simulink library "tqd"  (R2021b)
settings: Solver=VariableStepAuto  StartTime=0.0  StopTime=10.0  RelTol=1e-3
undefined symbols (not defined in the file): ATQD_AfterTqMinGain_X_Deg, ATQD_APSCreepBaseTqD_X_kph, ATQD_APSCreepBaseTqD_Y_Deg, ATQD_APSCreepBaseTqR_X_kph, ATQD_APSCreepBaseTqR_Y_Deg, ATQD_APSCreepIterm_X_kph, ATQD_APSCreepIterm_Y_kph, ATQD_APSCreepPterm_X_kph, ATQD_APSCreepPterm_Y_kph, ATQD_APSDecReq_X_kph, ATQD_APSDecReq_Y_mps2, ATQD_APSDecReqCMD_X_kph, ATQD_APSDecReqTs_X_pct, ATQD_APSDecTimeGain_X_Deg, ATQD_APSDecTimeGain_Y_s, ATQD_APSReqLowSpd_X_Deg, ATQD_AutoHoldReleaseBPS_X_Deg, ATQD_AWDLoadTrqnsGain_X_kg, ATQD_AWDLoadTrqnsGain_Y_pct, ATQD_BOSEnBPSPosn_X_kph, ATQD_BOSMap_X_rpm, ATQD_BOSMap_Y_pct, ATQD_CreepBaseTqD_X_kph, ATQD_CreepBaseTqD_Y_Deg, ATQD_CreepBaseTqR_X_kph, ATQD_CreepBaseTqR_Y_Deg, ATQD_CreepBPSDisPosn_X_Deg, ATQD_CreepBPSDisPosnR_X_Deg, ATQD_CreepBPSEnPosn_X_Deg, ATQD_CreepBPSEnPosnR_X_Deg, ATQD_CreepDeltaTq_X_kph, ATQD_CreepIterm_X_kph, ATQD_CreepIterm_Y_kph, ATQD_CreepItermMaxLimit_X_pct, ATQD_CreepPreloadTime_X_kph, ATQD_CreepPreloadTq_X_kph, ATQD_CreepPreloadTq_Y_s, ATQD_CreepProtTq_X_Deg, ATQD_CreepPterm_X_kph, ATQD_CreepPterm_Y_kph, ATQD_CreepRrTqSpRat_X_rpm, ATQD_CreepRrTqSpRat_Y_Nm, ATQD_CreepTargetSpdD_X_pct, ATQD_CreepTargetSpdR_X_pct, ATQD_ECOTqMapD_X_rpm, ATQD_ECOTqMapD_Y_pct, ATQD_EMTqMapD_X_rpm, ATQD_EMTqMapD_Y_pct, ATQD_EOPDTqMapDCon_X_rpm, ATQD_EOPDTqMapDCon_Y_Deg, ATQD_EscapeModePedTq_X_pct, ATQD_EscapeModePedTq_Y_rpm, ATQD_EscapeModePedTqFr_X_pct, ATQD_EscapeModePedTqFr_Y_rpm, ATQD_EstInitVehWeight_X_c, ATQD_FAfterTqCMDGain_X_rpm, ATQD_FAfterTqCMDGain_Y_pct, ATQD_FrLossMAPLowV_X_rpm, ATQD_FrLossMAPLowV_Y_Nm, ATQD_FrMotActReduce_X_rpm ... (+772)
libraries: simulink x211, hcu_lib x179, tqr x3
(part 2 of 28)

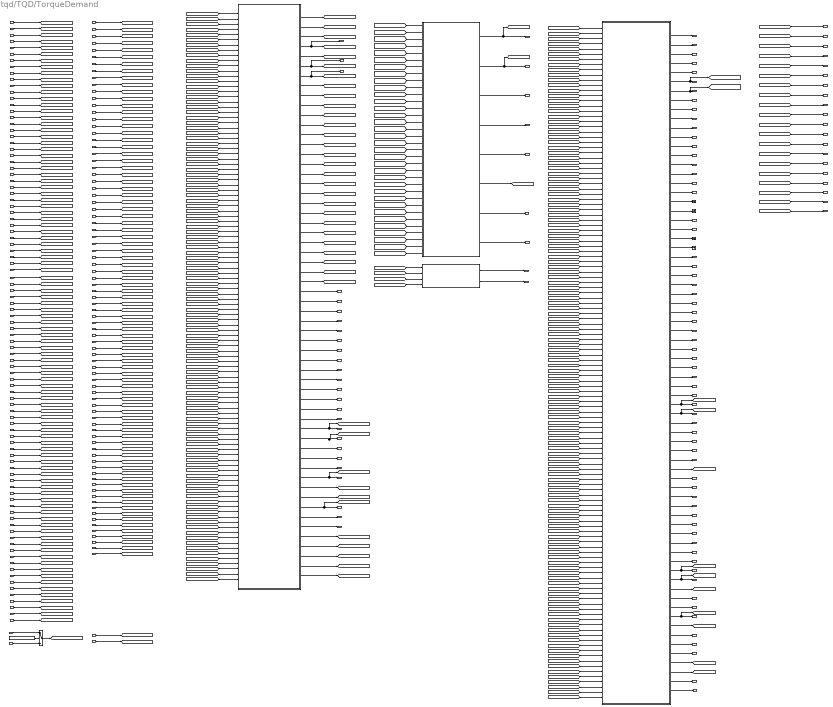
== system tqd/TQD/TorqueDemand ==
  note: Input Signals
  task_time_s : Inport
  VDHP_ActAPSPosn_pct : Inport  Port=2
  VDHP_LowIdleAccPedal_flg : Inport  Port=3
  VPMM_PowerSta_enum : Inport  Port=4
  VPMM_DrivetrainSelect_enum : Inport  Port=5
  VPMM_SysPowerMode_enum : Inport  Port=6
  VINP_VehSpeed_kph : Inport  Port=7
  VINP_BrkSwSta_flg : Inport  Port=8
  VINP_BrkSwV_flg : Inport  Port=9
  VINP_BrkPedalPos_pct : Inport  Port=10
  VINP_BrkPedalPosSta_flg : Inport  Port=11
  VINP_FrPTCSActive_flg : Inport  Port=12
  VINP_RrPTCSActive_flg : Inport  Port=13
  VINP_FrntAxlTrqReqDrv_Nm : Inport  Port=14
  VINP_RearAxlTrqReqDrv_Nm : Inport  Port=15
  VINP_FrRBCActive_flg : Inport  Port=16
  VINP_RrRBCActive_flg : Inport  Port=17
  VINP_FrntAxlTrqReqBrk_Nm : Inport  Port=18
  VINP_RearAxlTrqReqBrk_Nm : Inport  Port=19
  VINP_CrashOutputSts_enum : Inport  Port=20
  VINP_LongAccel_Gps : Inport  Port=21
  VINP_EPBCarWashMode_flg : Inport  Port=22
  VINP_EPBErrSta_enum : Inport  Port=23
  VINP_EPBSta_enum : Inport  Port=24
  VINP_DOASta_flg : Inport  Port=25
  VINP_GRADE_Deg : Inport  Port=26
  VINP_HSAActive_flg : Inport  Port=27
  VINP_DriverSeatBeltCmd_flg : Inport  Port=28
  VINP_AVHActive_flg : Inport  Port=29
  VINP_PsngrSeatBeltCmd_flg : Inport  Port=30
  VINP_RDriverSeatBeltCmd_flg : Inport  Port=31
  VINP_RCenterSeatBeltCmd_flg : Inport  Port=32
  VINP_RPsngrSeatBeltCmd_flg : Inport  Port=33
  VINP_YawRate_degps : Inport  Port=34
  VINP_SASAngle_Deg : Inport  Port=35
  VINP_ESCActive_flg : Inport  Port=36
  VINP_ABSActive_flg : Inport  Port=37
  VINP_LFRawWhlSpeed_kph : Inport  Port=38
  VINP_LRRawWhlSpeed_kph : Inport  Port=39
  VINP_RFRawWhlSpeed_kph : Inport  Port=40
  VINP_RRRawWhlSpeed_kph : Inport  Port=41
  VINP_ESCOFFStatus_enum : Inport  Port=42
  VINP_IVIPWModeReq_enum : Inport  Port=43
  VINP_IVICreepSWReq_flg : Inport  Port=44
  VINP_RollModeSWCmd_enum : Inport  Port=45
  VINP_IVIPwrLockSW_enum : Inport  Port=46
  VINP_IVIISAOffsetSpd_enum : Inport  Port=47
  VINP_Distanceunit_flg : Inport  Port=48
  VINP_SmartEcoModeSW_flg : Inport  Port=49
  VINP_IVISnowModeCmd_flg : Inport  Port=50
  VINP_IVIACCAdaptiveSta_flg : Inport  Port=51
  VINP_IVITrailerModeSWSta_flg : Inport  Port=52
  VINP_ShifterHandleCmd_enum : Inport  Port=53
  VINP_HVBPwrAvailDchrg_kw : Inport  Port=54
  VINP_HVBPwrAvailChrg_kw : Inport  Port=55
  VINP_HVBattErr_flg : Inport  Port=56
  VINP_DCDCFaultSta_enum : Inport  Port=57
  VINP_ChrgPlugSta_enum : Inport  Port=58
  VINP_HVBattSOC_pct : Inport  Port=59
  VINP_HVBattSOCDis_pct : Inport  Port=60
  VINP_HVBMTempMax_C : Inport  Port=61
  VINP_HVBMTempMin_C : Inport  Port=62
  VINP_ShifterFailsta_enum : Inport  Port=63
  VINP_FrEDURotateDirction_enum : Inport  Port=64
  VINP_RrEDURotateDirction_enum : Inport  Port=65
  VINP_FrTMSpd_RPM : Inport  Port=66
  VINP_RrTMSpd_RPM : Inport  Port=67
  VINP_FrRegenAvailTq_Nm : Inport  Port=68
  VINP_RrRegenAvailTq_Nm : Inport  Port=69
  VINP_FrEDURealTMTq_Nm : Inport  Port=70
  VINP_RrEDURealTMTq_Nm : Inport  Port=71
  VINP_FrMotorAvailTq_Nm : Inport  Port=72
  VINP_RrMotorAvailTq_Nm : Inport  Port=73
  VINP_MCUWarnF_enum : Inport  Port=74
  VINP_MCUWarnR_enum : Inport  Port=75
  VINP_FrMCUDCBusVolt_V : Inport  Port=76
  VINP_RrMCUDCBusVolt_V : Inport  Port=77
  VINP_FrMCUTemp_C : Inport  Port=78
  VINP_FrTMTemp_C : Inport  Port=79
  VINP_RrMCUTemp_C : Inport  Port=80
  VINP_RrTMTemp_C : Inport  Port=81
  VINP_SWCResUpSta_flg : Inport  Port=82
  VINP_SWCSetdownSta_flg : Inport  Port=83
  VINP_SWCACCSta_flg : Inport  Port=84
  VINP_SWCCANCELSta_flg : Inport  Port=85
  VINP_SWC2LScrollUpSta_flg : Inport  Port=86
  VINP_SWC2LScrollDownSta_flg : Inport  Port=87
  VINP_SWC2LScrollPressSta_flg : Inport  Port=88
  VINP_SWC2LADASSta_flg : Inport  Port=89
  VINP_SWC2RScrollPressSta_flg : Inport  Port=90
  VINP_SWC2RScrollUpSta_flg : Inport  Port=91
  VINP_SWC2RScrollDownSta_flg : Inport  Port=92
  VINP_SWC2LDriveModeSta_flg : Inport  Port=93
  VINP_SWC2RRightSta_flg : Inport  Port=94
  VINP_SWC2RLeftSta_flg : Inport  Port=95
  VINP_SWC2RCustomizeSta_flg : Inport  Port=96
  VINP_SWCRegenUp_flg : Inport  Port=97
  VINP_SWCRegenDown_flg : Inport  Port=98
  VINP_ADASForceIdle_flg : Inport  Port=99
  VVMC_ACCRequiredAccel_mps2 : Inport  Port=100
  VINP_ACCVehHoldReq_flg : Inport  Port=101
  VVMC_ADASActive_flg : Inport  Port=102
  VVMC_ADASWhlTqReq_Nm : Inport  Port=103
  VVMC_CruzActive_flg : Inport  Port=104
  VVMC_CruzWhlTqReq_Nm : Inport  Port=105
  VVMC_MSAActive_flg : Inport  Port=106
  VVMC_MSAWhlTqReq_Nm : Inport  Port=107
  VVMC_APSActive_flg : Inport  Port=108
  VVMC_APSSpeedCMD_kph : Inport  Port=109
  VVMC_APSShiftPosnReq_enum : Inport  Port=110
  VVMC_ACCPedalOvrd_flg : Inport  Port=111
  VVMC_LongAcc_Gps : Inport  Port=112
  VVMC_ActMaxSlideRate_pct : Inport  Port=113
  VVMC_EstSlope_Deg : Inport  Port=114
  VVMC_APSReq_enum : Inport  Port=115
  VVMC_RWDRDCActive_enum : Inport  Port=116
  VVMC_ActLRSlideRate_pct : Inport  Port=117
  VVMC_ActRRSlideRate_pct : Inport  Port=118
  VVMC_ActStESCYaw_degps : Inport  Port=119
  VVMC_CCCtrlSta_enum : Inport  Port=120
  VVMC_MSACtrlSta_enum : Inport  Port=121
  VVMC_LVDAACCStatusInformation_flg : Inport  Port=122
  VVMC_ACCObjDist_m : Inport  Port=123
  VVMC_MeterIndSpeed_raw32 : Inport  Port=124
  VVMC_RearTqRatio_rat : Inport  Port=125
  VVMC_CalibratedGyroY_Dps : Inport  Port=126
  VVMC_CAASActive_flg : Inport  Port=127
  VVMC_SetACCDisableAPS_flg : Inport  Port=128
  VINP_BrakeSWGPIO_flg : Inport  Port=129
  VINP_CrashSignalGPIO_flg : Inport  Port=130
  VINP_DrDoorSW_flg : Inport  Port=131
  VINP_SeatSW_flg : Inport  Port=132
  VINP_HoodSW_flg : Inport  Port=133
  VINP_TailgateSW_flg : Inport  Port=134
  VINP_PsDoorSW_flg : Inport  Port=135
  VINP_RRDoorSW_flg : Inport  Port=136
  VINP_RLDoorSW_flg : Inport  Port=137
  VTQR_ActualFEDUWhlTqReq_Nm : Inport  Port=138
  VTQR_ActualREDUWhlTqReq_Nm : Inport  Port=139
  VTQR_NoABSFEDUWhlTqReq_Nm : Inport  Port=140
  VTQR_NoABSREDUWhlTqReq_Nm : Inport  Port=141
  VTQR_RShaftSpdTqLimLow_flg : Inport  Port=142
  VTQR_RTimerTqLimLow_flg : Inport  Port=143
  VTQR_FShaftSpdTqLimLow_flg : Inport  Port=144
  VTQR_FTimerTqLimLow_flg : Inport  Port=145
  VTQR_FrFirstOrderInpTs_c : Inport  Port=146
  VTQR_RrFirstOrderInpTs_c : Inport  Port=147
  VTQR_FrRateLimitInc_Nm : Inport  Port=148
  VTQR_FrRateLimitDec_Nm : Inport  Port=149
  VTQR_RrRateLimitInc_Nm : Inport  Port=150
  VTQR_RrRateLimitDec_Nm : Inport  Port=151
  VTQR_FrTqZeroTransLowBound_Nm : Inport  Port=152
  VTQR_RrTqZeroTransUpBound_Nm : Inport  Port=153
  VINP_PBWMotorPos_enum : Inport  Port=154
  VBCM_BrakeLamp_flg : Inport  Port=155
  VBCM_UserNow_enum : Inport  Port=156
  VINP_ADASISASta_enum : Inport  Port=157
  VINP_ADASVehSpdLim_kph : Inport  Port=158
  VINP_ADASACCSta_enum : Inport  Port=159
  VINP_ADASSLIFSpdLim_enum : Inport  Port=160
  VINP_ADASAEBSta_enum : Inport  Port=161
  VINP_FlashRegenMode_enum : Inport  Port=162
  VINP_VehicleType_enum : Inport  Port=163
  VINP_SWCType_enum : Inport  Port=164
  VINP_CAASSta_enum : Inport  Port=165
  VINP_APSStaSystem_enum : Inport  Port=166
  VBCM_RegenModeUserSetting_enum : Inport  Port=167
  VINP_IVIEscapeModeCmd_flg : Inport  Port=168
  VDDM_VCURAPSErrLv2_flg : Inport  Port=169
  VDDM_VCURAPSErrLv3_flg : Inport  Port=170
  VDDM_EPBSigErrCFS_flg : Inport  Port=171
  VDDM_EPB1Err_flg : Inport  Port=172
  VDDM_ESC1Err_flg : Inport  Port=173
  VDDM_ESC5Err_flg : Inport  Port=174
  VDDM_LimpHomeAct_flg : Inport  Port=175
  VDDM_VehMalfunLevel_enum : Inport  Port=176
  VDDM_Shifter1Err_flg : Inport  Port=177
  VDDM_ShifterSigErrCFS_flg : Inport  Port=178
  VDDM_MCUF1Err_flg : Inport  Port=179
  VDDM_MCUR1Err_flg : Inport  Port=180
  VDDM_RegenErrCFS_flg : Inport  Port=181
  VDDM_4D2CErr_flg : Inport  Port=182
  Constant21 : Constant  Value=KTQD_YawRateSW_flg
  CrashDetect : Subsystem
  ShiftModule : Subsystem
      settings: AttributesFormatString=Priority%<Priority>
  Signal_convert : Subsystem
  Switch : Switch  Criteria=u2 > Threshold
  Terminator{,1..3} (4 alike) : Terminator
  TorqueModule : Subsystem
      settings: AttributesFormatString=Priority%<Priority>
  VTQD_GearActualPosn_enum : Outport
  VTQD_ParkRequest_flg : Outport  Port=2
  VTQD_PBWLockTO_flg : Outport  Port=3
  VTQD_PBWUnlockTO_flg : Outport  Port=4
  VTQD_DriverWhlTqDem_Nm : Outport  Port=5
  VTQD_AfterAvailableTqDemFr_Nm : Outport  Port=6
  VTQD_AfterAvailableTqDemRr_Nm : Outport  Port=7
  VTQD_TqSourceFr_enum : Outport  Port=8
  VTQD_TqSourceRr_enum : Outport  Port=9
  VTQD_FrEDUAvailBrkRgnTq_Nm : Outport  Port=10
  VTQD_RrEDUAvailBrkRgnTq_Nm : Outport  Port=11
  VTQD_TqTargetShaftSpd_rpm : Outport  Port=12
  VTQD_LimpHomeAct_flg : Outport  Port=13
  VTQD_RollRegenEnable_flg : Outport  Port=14
  VTQD_EVDriveMode_enum : Outport  Port=15
  VTQD_EVDriveModeValid_flg : Outport  Port=16
  VTQD_ShiftGearPosn_enum : Outport  Port=17
  VTQD_PButtonSta_enum : Outport  Port=18
  VTQD_FrActvDmpDisabReq_flg : Outport  Port=19
  VTQD_RrActvDmpDisabReq_flg : Outport  Port=20
  VTQD_FrRgnDecrSta_flg : Outport  Port=21
  VTQD_RrRgnDecrSta_flg : Outport  Port=22
  VTQD_DriverWhlTqDemFr_Nm : Outport  Port=23
  VTQD_DriverWhlTqDemRr_Nm : Outport  Port=24
  VTQD_FrEDUActTq_Nm : Outport  Port=25
  VTQD_RrEDUActTq_Nm : Outport  Port=26
  VTQD_FrEDURolRgnTq_Nm : Outport  Port=27
  VTQD_RrEDURolRgnTq_Nm : Outport  Port=28
  VTQD_FrEDUSpd_rpm : Outport  Port=29
  VTQD_RrEDUSpd_rpm : Outport  Port=30
  VTQD_FrEDUSpdValid_flg : Outport  Port=31
  VTQD_FrEDUAvailBrkRgnTqV_flg : Outport  Port=32
  VTQD_RrEDUSpdValid_flg : Outport  Port=33
  VTQD_RrEDUAvailBrkRgnTqV_flg : Outport  Port=34
  VTQD_RgnAbnorSta_flg : Outport  Port=35
  VTQD_PTCSPermSta_flg : Outport  Port=36
  VTQD_FrRgnPermSta_flg : Outport  Port=37
  VTQD_RrRgnPermSta_flg : Outport  Port=38
  VTQD_ExternalTqAllow_flg : Outport  Port=39
  VTQD_FrIdcMin_A : Outport  Port=40
  VTQD_FrIdcMax_A : Outport  Port=41
  VTQD_FrUdcMin_V : Outport  Port=42
  VTQD_FrUdcMax_V : Outport  Port=43
  VTQD_RrIdcMin_A : Outport  Port=44
  VTQD_RrIdcMax_A : Outport  Port=45
  VTQD_RrUdcMin_V : Outport  Port=46
  VTQD_RrUdcMax_V : Outport  Port=47
  VTQD_CoordWhlTqDemFr_Nm : Outport  Port=48
  VTQD_CoordWhlTqDemRr_Nm : Outport  Port=49
  VTQD_CreepEnable_flg : Outport  Port=50
  VTQD_CrashDetd_flg : Outport  Port=51
  VTQD_DiagHCrash_flg : Outport  Port=52
  VTQD_ReBrakeLPReq_flg : Outport  Port=53
  VTQD_LoSpdBrkCtrl_flg : Outport  Port=54
  VTQD_LowIdleAccPedal_flg : Outport  Port=55
  VTQD_APSStaSys_enum : Outport  Port=56
  VTQD_APSReq_enum : Outport  Port=57
  VTQD_APSDecReqA_flg : Outport  Port=58
  VTQD_APSDecReq_mps2 : Outport  Port=59
  VTQD_ExtShftAllow_flg : Outport  Port=60
  VTQD_EstVehWeightResult_kg : Outport  Port=61
  VTQD_BOSEnable_flg : Outport  Port=62
  VTQD_CreepON_flg : Outport  Port=63
  VTQD_PreLoadHold_flg : Outport  Port=64
  VTQD_PreLoadPreEn_flg : Outport  Port=65
  VTQD_CreepPrLoadEnable_flg : Outport  Port=66
  VTQD_RDCActive_enum : Outport  Port=67
  VTQD_EquivAccPedalSWSta_flg : Outport  Port=68
  VTQD_DriveProtEn_flg : Outport  Port=69
  VTQD_ActParkRequest_flg : Outport  Port=70
  VTQD_RegenTqLimitEn_flg : Outport  Port=71
  VTQD_PedAccTqEn_flg : Outport  Port=72
  VTQD_IVIPwrLockSta_enum : Outport  Port=73
  VTQD_ExtDoorAllow_flg : Outport  Port=74
  VTQD_WhlTqCapGenFr_Nm : Outport  Port=75
  VTQD_WhlTqCapGenRr_Nm : Outport  Port=76
  VTQD_OPDHoldLamp_flg : Outport  Port=77
  VTQD_RegenMode_enum : Outport  Port=78
  VTQD_SaveRegenMode_enum : Outport  Port=79
  VTQD_FDCVCURegenMode_enum : Outport  Port=80
  VTQD_SpdCtrlMode_enum : Outport  Port=81
  VTQD_SpdCtrlSta_flg : Outport  Port=82
  VTQD_SetSpd_kph : Outport  Port=83
  VTQD_SWCCancelSta_flg : Outport  Port=84
  VTQD_SWCSetdownSta_flg : Outport  Port=85
  VTQD_SWCResUpSta_flg : Outport  Port=86
  VTQD_CreepBaseTqD_Nm : Outport  Port=87
  VTQD_VehActSpd_kph : Outport  Port=88
  VTQD_RegenLimIndSta_flg : Outport  Port=89
  VTQD_BrkSwSta_flg : Outport  Port=90
  VTQD_SWC2CancelSta_flg : Outport  Port=91
  VTQD_SWC2SetdownSta_flg : Outport  Port=92
  VTQD_SWC2ResUpSta_flg : Outport  Port=93
  VTQD_SWC2LADASSta_flg : Outport  Port=94
  VTQD_SpdLim4SetSpd_raw32 : Outport  Port=95
  VTQD_SetSpdLimWarn_flg : Outport  Port=96
  VTQD_MaxWhlSlideRate_pct : Outport  Port=97
  VTQD_MinWhlSlideRate_pct : Outport  Port=98
  VTQD_LeftSlideRate_pct : Outport  Port=99
  VTQD_RightSlideRate_pct : Outport  Port=100
  VTQD_FrontSlideRate_pct : Outport  Port=101
  VTQD_RearSlideRate_pct : Outport  Port=102
  VTQD_TrailerDisOPDSta_flg : Outport  Port=103
  VTQD_ComboKeyPreEn_flg : Outport  Port=104
  VTQD_ComboKeyEn_flg : Outport  Port=105
  VTQD_SysMode_enum : Outport  Port=106
  VTQD_WhlTqCapMotFr_Nm : Outport  Port=107
  VTQD_WhlTqCapMotRr_Nm : Outport  Port=108
  VTQD_FrShaftSpd_rpm : Outport  Port=109
  VTQD_RrShaftSpd_rpm : Outport  Port=110
  VTQD_EPBCarWashMode_flg : Outport  Port=111
  VTQD_IVIRockModeEn_flg : Outport  Port=112
  VTQD_ForceP_flg : Outport  Port=113
  VTQD_SlideRegenLimTq_Nm : Outport  Port=114
  VTQD_SimSoundCmd_pct : Outport  Port=115
  VTQD_SimSouWaveReq_pct : Outport  Port=116
  VTQD_RockModeTCSReq_flg : Outport  Port=117
  VTQD_TMEnOutpTqSta_enum : Outport  Port=118
  wires:
  VINP_FrTMSpd_RPM/1 -> [VINP_FrTMSpd_rpm]
  VDHP_ActAPSPosn_pct/1 -> [VDHP_ActAPSPosn_pct]
  VPMM_PowerSta_enum/1 -> [VPMM_PowerSta_enum]
  task_time_s/1 -> [task_time_s]
  VINP_VehSpeed_kph/1 -> [VINP_VehSpeed_kph]
  VINP_BrkSwSta_flg/1 -> [VINP_BrkSwSta_flg]
  VINP_ShifterHandleCmd_enum/1 -> [VINP_ShifterHandleCmd_enum]
  VDHP_LowIdleAccPedal_flg/1 -> [VDHP_LowIdleAccPedal_flg]
  VINP_PBWMotorPos_enum/1 -> [VINP_PBWMotorPos_enum]
  Signal_convert/8(VTQD_TqTargetShaftSpd_rpm) -> [VTQD_TqTargetShaftSpd_rpm]
  Signal_convert/2(VTQD_RollRegenDisable_flg) -> [VTQD_RollRegenDisableReq_flg]
  Signal_convert/5(VTQD_ActBPSPosn_pct) -> [VTQD_ActBPSPosn_pct]
  Signal_convert/11(VTQD_EVDriveMode_enum) -> [VTQD_EVDriveMode_enum]
  Signal_convert/10(VTQD_LimpHomeAct_flg) -> [VTQD_LimpHomeAct_flg]
  Signal_convert/12(VTQD_CreepON_flg) -> [VTQD_CreepON_flg]
  [VTQD_TMRotateDirction_enum] -> ShiftModule/7(VTQD_TMRotateDirction_enum)
  ShiftModule/4(VTQD_PBWUnlockTO_flg) -> VTQD_PBWUnlockTO_flg/1
  [VTQD_VehActSpd_kph] -> ShiftModule/3(VTQD_VehActSpd_kph)
  [VPMM_PowerSta_enum] -> ShiftModule/5(VPMM_PowerSta_enum)
  [task_time_s] -> ShiftModule/1(task_time_s)
  [VTQD_BrkSwSta_flg] -> ShiftModule/4(VTQD_BrkSwSta_flg)
  ShiftModule/2(VTQD_ParkRequest_flg) -> [VTQD_ParkRequest_flg], VTQD_ParkRequest_flg/1
  [VTQD_ShifterHandleCmd_enum] -> ShiftModule/2(VTQD_ShifterHandleCmd_enum)
  ShiftModule/3(VTQD_PBWLockTO_flg) -> VTQD_PBWLockTO_flg/1
  [VINP_PBWMotorPos_enum] -> ShiftModule/6(VINP_PBWMotorPos_enum)
  ShiftModule/1(VTQD_GearActualPosn_enum) -> VTQD_GearActualPosn_enum/1, [VTQD_GearActualPosn_enum]
  [VTQD_RollRegenDisableReq_flg] -> TorqueModule/3(VTQD_RollRegenDisableReq_flg)
  [VTQD_GearActualPosn_enum] -> TorqueModule/4(VTQD_GearActualPosn_enum)
  [VTQD_CreepON_flg] -> TorqueModule/5(VTQD_CreepON_flg)
  [VTQD_BrkSwSta_flg] -> TorqueModule/6(VTQD_BrkSwSta_flg)
  [VINP_FrntAxlTrqReqBrk_Nm] -> TorqueModule/22(VINP_FrntAxlTrqReqBrk_Nm)
  [VINP_RearAxlTrqReqBrk_Nm] -> TorqueModule/23(VINP_RearAxlTrqReqBrk_Nm)
  [VINP_RearAxlTrqReqDrv_Nm] -> TorqueModule/19(VINP_RearAxlTrqReqDrv_Nm)
  [VINP_FrntAxlTrqReqDrv_Nm] -> TorqueModule/18(VINP_FrntAxlTrqReqDrv_Nm)
  [VTQD_LimpHomeAct_flg] -> TorqueModule/7(VTQD_LimpHomeAct_flg)
  [VINP_VehSpeed_kph] -> TorqueModule/10(VINP_VehSpeed_kph)
  [VTQD_TqTargetShaftSpd_rpm] -> TorqueModule/11(VTQD_TqTargetShaftSpd_rpm)
  [VTQD_ActBPSPosn_pct] -> TorqueModule/15(VTQD_ActBPSPosn_pct)
  [VVMC_APSActive_flg] -> TorqueModule/30(VVMC_APSActive_flg)
  [VVMC_ADASActive_flg] -> TorqueModule/24(VVMC_ADASActive_flg)
  [VVMC_ADASWhlTqReq_Nm] -> TorqueModule/25(VVMC_ADASWhlTqReq_Nm)
  [VVMC_CruzActive_flg] -> TorqueModule/26(VVMC_CruzActive_flg)
  [VVMC_CruzWhlTqReq_Nm] -> TorqueModule/27(VVMC_CruzWhlTqReq_Nm)
  [VVMC_MSAActive_flg] -> TorqueModule/28(VVMC_MSAActive_flg)
  [VVMC_MSAWhlTqReq_Nm] -> TorqueModule/29(VVMC_MSAWhlTqReq_Nm)
  VINP_HVBPwrAvailDchrg_kw/1 -> [VINP_HVBPwrAvailDchrg_kw]
  VINP_HVBPwrAvailChrg_kw/1 -> [VINP_HVBPwrAvailChrg_kw]
  [VINP_HVBPwrAvailDchrg_kw] -> TorqueModule/31(VINP_HVBPwrAvailDchrg_kw)
  [VINP_HVBPwrAvailChrg_kw] -> TorqueModule/34(VINP_HVBPwrAvailChrg_kw)
  VDDM_LimpHomeAct_flg/1 -> [VDDM_LimpHomeAct_flg]
  [VDDM_LimpHomeAct_flg] -> Signal_convert/14(VDDM_LimpHomeAct_flg)
  VINP_BrkSwV_flg/1 -> [VINP_BrkSwV_flg]
  VINP_FrPTCSActive_flg/1 -> [VINP_FrPTCSActive_flg]
  VINP_FrntAxlTrqReqDrv_Nm/1 -> [VINP_FrntAxlTrqReqDrv_Nm]
  VINP_RearAxlTrqReqDrv_Nm/1 -> [VINP_RearAxlTrqReqDrv_Nm]
  VINP_FrRBCActive_flg/1 -> [VINP_FrRBCActive_flg]
  VINP_FrntAxlTrqReqBrk_Nm/1 -> [VINP_FrntAxlTrqReqBrk_Nm]
  VINP_RearAxlTrqReqBrk_Nm/1 -> [VINP_RearAxlTrqReqBrk_Nm]
  VINP_BrkPedalPos_pct/1 -> [VINP_BrkPedalPos_pct]
  VINP_BrkPedalPosSta_flg/1 -> [VINP_BrkPedalPosSta_flg]
  [VINP_BrkSwSta_flg] -> Signal_convert/4(VINP_BrkSwSta_flg)
  [VINP_BrkSwV_flg] -> Signal_convert/6(VINP_BrkSwV_flg)
  [VINP_BrkPedalPos_pct] -> Signal_convert/7(VINP_BrkPedalPos_pct)
  [VINP_BrkPedalPosSta_flg] -> Signal_convert/8(VINP_BrkPedalPosSta_flg)
  [VTQD_TqTargetShaftSpd_rpm] -> VTQD_TqTargetShaftSpd_rpm/1
  [VTQD_LowIdleAccPedal_flg] -> TorqueModule/1(VTQD_LowIdleAccPedal_flg)
  [VPMM_DrivetrainSelect_enum] -> TorqueModule/2(VPMM_DrivetrainSelect_enum)
  VINP_RrTMSpd_RPM/1 -> [VINP_RrTMSpd_rpm]
  [VPMM_DrivetrainSelect_enum] -> Signal_convert/11(VPMM_DrivetrainSelect_enum)
  VPMM_DrivetrainSelect_enum/1 -> [VPMM_DrivetrainSelect_enum]
  [VDHP_ActAPSPosn_pct] -> Signal_convert/3(VDHP_ActAPSPosn_pct)
  Signal_convert/3(VTQD_ActAPSPosn_pct) -> [VTQD_ActAPSPosn_pct]
  [VTQD_ActAPSPosn_pct] -> TorqueModule/14(VTQD_ActAPSPosn_pct)
  [VTQD_GearActualPosn_enum] -> Signal_convert/1(VTQD_GearActualPosn_enum)
  [VINP_FrTMSpd_rpm] -> Signal_convert/9(VINP_FrTMSpd_rpm)
  [VINP_RrTMSpd_rpm] -> Signal_convert/10(VINP_RrTMSpd_rpm)
  VINP_FrEDURotateDirction_enum/1 -> [VINP_FrEDURotateDirction_enum]
  VINP_RrEDURotateDirction_enum/1 -> [VINP_RrEDURotateDirction_enum]
  [VINP_RrEDURotateDirction_enum] -> Signal_convert/13(VINP_RrEDURotateDirction_enum)
  [VINP_FrEDURotateDirction_enum] -> Signal_convert/12(VINP_FrEDURotateDirction_enum)
  Signal_convert/6(VTQD_FrShaftSpd_rpm) -> VTQD_FrShaftSpd_rpm/1, [VTQD_FrShaftSpd_rpm]
  Signal_convert/7(VTQD_RrShaftSpd_rpm) -> VTQD_RrShaftSpd_rpm/1, [VTQD_RrShaftSpd_rpm]
  Signal_convert/9(VTQD_TMRotateDirction_enum) -> [VTQD_TMRotateDirction_enum]
  Signal_convert/4(VTQD_BrkSwSta_flg) -> [VTQD_BrkSwSta_flg], VTQD_BrkSwSta_flg/1
  [VTQD_FrShaftSpd_rpm] -> TorqueModule/12(VTQD_FrShaftSpd_rpm)
  [VTQD_RrShaftSpd_rpm] -> TorqueModule/13(VTQD_RrShaftSpd_rpm)
  Signal_convert/1(VTQD_LowIdleAccPedal_flg) -> [VTQD_LowIdleAccPedal_flg]
  [VDHP_LowIdleAccPedal_flg] -> Signal_convert/2(VDHP_LowIdleAccPedal_flg)
  [VTQD_LimpHomeAct_flg] -> VTQD_LimpHomeAct_flg/1
  [VTQD_EVDriveMode_enum] -> VTQD_EVDriveMode_enum/1
  VINP_BrakeSWGPIO_flg/1 -> [VINP_BrakeSWGPIO_flg]
  [VINP_BrakeSWGPIO_flg] -> Signal_convert/5(VINP_BrakeSWGPIO_flg)
  Signal_convert/13(VTQD_ShiftGearPosn_enum) -> [VTQD_ShiftGearPosn_enum]
  [VTQD_ShiftGearPosn_enum] -> VTQD_ShiftGearPosn_enum/1
  ShiftModule/5(VTQD_PButtonSta_enum) -> VTQD_PButtonSta_enum/1
  [VINP_VehSpeed_kph] -> Signal_convert/15(VINP_VehSpeed_kph)
  Signal_convert/14(VTQD_FrActvDmpDisabReq_flg) -> [VTQD_FrActvDmpDisabReq_flg]
  Signal_convert/15(VTQD_RrActvDmpDisabReq_flg) -> [VTQD_RrActvDmpDisabReq_flg]
  [VTQD_FrActvDmpDisabReq_flg] -> VTQD_FrActvDmpDisabReq_flg/1
  [VTQD_RrActvDmpDisabReq_flg] -> VTQD_RrActvDmpDisabReq_flg/1
  VINP_RrPTCSActive_flg/1 -> [VINP_RrPTCSActive_flg]
  [VINP_FrPTCSActive_flg] -> TorqueModule/16(VINP_FrPTCSActive_flg)
  [VINP_RrPTCSActive_flg] -> TorqueModule/17(VINP_RrPTCSActive_flg)
  VINP_RrRBCActive_flg/1 -> [VINP_RrRBCActive_flg]
  [VINP_FrRBCActive_flg] -> TorqueModule/20(VINP_FrRBCActive_flg)
  [VINP_RrRBCActive_flg] -> TorqueModule/21(VINP_RrRBCActive_flg)
  VINP_RrRegenAvailTq_Nm/1 -> [VINP_RrRegenAvailTq_Nm]
  VINP_FrEDURealTMTq_Nm/1 -> [VINP_FrEDURealTMTq_Nm]
  VINP_FrRegenAvailTq_Nm/1 -> [VINP_FrRegenAvailTq_Nm]
  VINP_RrEDURealTMTq_Nm/1 -> [VINP_RrEDURealTMTq_Nm]
  [VINP_FrRegenAvailTq_Nm] -> TorqueModule/35(VINP_FrRegenAvailTq_Nm)
  [VINP_RrRegenAvailTq_Nm] -> TorqueModule/36(VINP_RrRegenAvailTq_Nm)
  [VINP_FrTMSpd_rpm] -> TorqueModule/37(VINP_FrTMSpd_RPM)
  [VINP_RrTMSpd_rpm] -> TorqueModule/38(VINP_RrTMSpd_RPM)
  [VINP_FrEDURealTMTq_Nm] -> TorqueModule/39(VINP_FrEDURealTMTq_Nm)
  [VINP_RrEDURealTMTq_Nm] -> TorqueModule/40(VINP_RrEDURealTMTq_Nm)
  [VTQD_ParkRequest_flg] -> TorqueModule/41(VTQD_ParkRequest_flg)
  Signal_convert/16(VTQD_MCUReady4Ext_flg) -> [VTQD_MCUReady4Ext_flg]
  [VPMM_PowerSta_enum] -> TorqueModule/42(VPMM_PwrSta_enum)
  [VTQD_MCUReady4Ext_flg] -> TorqueModule/43(VTQD_MCUReady4Ext_flg)
  VINP_DCDCFaultSta_enum/1 -> [VINP_DCDCFaultSta_enum]
  VINP_ADASForceIdle_flg/1 -> [VINP_ADASForceIdle_flg]
  VINP_HVBattErr_flg/1 -> [VINP_HVBattErr_flg]
  [VINP_HVBattErr_flg] -> TorqueModule/44(VINP_HVBattErr_flg)
  [VINP_DCDCFaultSta_enum] -> TorqueModule/45(VINP_DCDCFaultSta_enum)
  [VINP_ADASForceIdle_flg] -> TorqueModule/46(VINP_ADASForceIdle_flg)
  VVMC_ADASActive_flg/1 -> [VVMC_ADASActive_flg]
  VVMC_ADASWhlTqReq_Nm/1 -> [VVMC_ADASWhlTqReq_Nm]
  VVMC_APSActive_flg/1 -> [VVMC_APSActive_flg]
  [VTQD_TMRotateDirction_enum] -> TorqueModule/47(VTQD_TMRotateDirction_enum)
  VINP_IVIPWModeReq_enum/1 -> [VINP_IVIPWModeReq_enum]
  [VTQD_EVDriveMode_enum] -> TorqueModule/8(VTQD_EVDriveMode_enum)
  [VTQD_RegenMode_enum] -> TorqueModule/9(VTQD_RegenMode_enum)
  TorqueModule/1(VTQD_DriverWhlTqDem_Nm) -> VTQD_DriverWhlTqDem_Nm/1
  TorqueModule/2(VTQD_TqSourceFr_enum) -> VTQD_TqSourceFr_enum/1
  TorqueModule/3(VTQD_TqSourceRr_enum) -> VTQD_TqSourceRr_enum/1  "VTQD_TqSourceRr_enum"
  TorqueModule/4(VTQD_RollRegenEnable_flg) -> VTQD_RollRegenEnable_flg/1
  TorqueModule/5(VTQD_EVDriveModeValid_flg) -> VTQD_EVDriveModeValid_flg/1
  TorqueModule/7(VTQD_AfterAvailableTqDemRr_Nm) -> [VTQD_AfterAvailableTqDemRr_Nm], VTQD_AfterAvailableTqDemRr_Nm/1
  TorqueModule/8(VTQD_FrEDUAvailBrkRgnTq_Nm) -> VTQD_FrEDUAvailBrkRgnTq_Nm/1
  TorqueModule/9(VTQD_RrEDUAvailBrkRgnTq_Nm) -> VTQD_RrEDUAvailBrkRgnTq_Nm/1
  TorqueModule/10(VTQD_FrRgnDecrSta_flg) -> VTQD_FrRgnDecrSta_flg/1
  TorqueModule/11(VTQD_RrRgnDecrSta_flg) -> VTQD_RrRgnDecrSta_flg/1
  TorqueModule/12(VTQD_FrEDUActTq_Nm) -> VTQD_FrEDUActTq_Nm/1
  TorqueModule/13(VTQD_RrEDUActTq_Nm) -> VTQD_RrEDUActTq_Nm/1
  TorqueModule/14(VTQD_FrEDURolRgnTq_Nm) -> VTQD_FrEDURolRgnTq_Nm/1
  TorqueModule/15(VTQD_RrEDURolRgnTq_Nm) -> VTQD_RrEDURolRgnTq_Nm/1
  TorqueModule/16(VTQD_FrEDUSpd_rpm) -> VTQD_FrEDUSpd_rpm/1
  TorqueModule/17(VTQD_RrEDUSpd_rpm) -> VTQD_RrEDUSpd_rpm/1
  TorqueModule/18(VTQD_FrEDUSpdValid_flg) -> VTQD_FrEDUSpdValid_flg/1
  TorqueModule/21(VTQD_FrEDUAvailBrkRgnTqV_flg) -> VTQD_FrEDUAvailBrkRgnTqV_flg/1
  TorqueModule/22(VTQD_RrEDUSpdValid_flg) -> VTQD_RrEDUSpdValid_flg/1
  TorqueModule/23(VTQD_RrEDUActTqValid_flg) -> Terminator2/1
  TorqueModule/24(VTQD_RrEDURolRgnTqValid_flg) -> Terminator3/1
  TorqueModule/25(VTQD_RrEDUAvailBrkRgnTqV_flg) -> VTQD_RrEDUAvailBrkRgnTqV_flg/1
  TorqueModule/26(VTQD_RgnAbnorSta_flg) -> VTQD_RgnAbnorSta_flg/1
  TorqueModule/27(VTQD_PTCSPermSta_flg) -> VTQD_PTCSPermSta_flg/1
  TorqueModule/28(VTQD_FrRgnPermSta_flg) -> VTQD_FrRgnPermSta_flg/1
  TorqueModule/29(VTQD_RrRgnPermSta_flg) -> VTQD_RrRgnPermSta_flg/1
  TorqueModule/30(VTQD_DriverWhlTqDemFr_Nm) -> VTQD_DriverWhlTqDemFr_Nm/1
  TorqueModule/31(VTQD_DriverWhlTqDemRr_Nm) -> VTQD_DriverWhlTqDemRr_Nm/1
  TorqueModule/32(VTQD_ExternalTqAllow_flg) -> VTQD_ExternalTqAllow_flg/1
  TorqueModule/33(VTQD_FrIdcMin_A) -> VTQD_FrIdcMin_A/1
  TorqueModule/34(VTQD_FrIdcMax_A) -> VTQD_FrIdcMax_A/1
  TorqueModule/35(VTQD_FrUdcMin_V) -> VTQD_FrUdcMin_V/1
  TorqueModule/36(VTQD_FrUdcMax_V) -> VTQD_FrUdcMax_V/1
  TorqueModule/37(VTQD_RrIdcMin_A) -> VTQD_RrIdcMin_A/1
  TorqueModule/38(VTQD_RrIdcMax_A) -> VTQD_RrIdcMax_A/1
  TorqueModule/39(VTQD_RrUdcMin_V) -> VTQD_RrUdcMin_V/1
  TorqueModule/40(VTQD_RrUdcMax_V) -> VTQD_RrUdcMax_V/1
  TorqueModule/41(VTQD_CoordWhlTqDemFr_Nm) -> VTQD_CoordWhlTqDemFr_Nm/1, [VTQD_CoordWhlTqDemFr_Nm]
  TorqueModule/42(VTQD_CoordWhlTqDemRr_Nm) -> VTQD_CoordWhlTqDemRr_Nm/1, [VTQD_CoordWhlTqDemRr_Nm]
  TorqueModule/43(VTQD_CreepEnable_flg) -> VTQD_CreepEnable_flg/1
  [VINP_IVIPWModeReq_enum] -> Signal_convert/16(VINP_IVIPWModeReq_enum)
  VVMC_CruzActive_flg/1 -> [VVMC_CruzActive_flg]
  VVMC_CruzWhlTqReq_Nm/1 -> [VVMC_CruzWhlTqReq_Nm]
  VVMC_MSAActive_flg/1 -> [VVMC_MSAActive_flg]
  VVMC_MSAWhlTqReq_Nm/1 -> [VVMC_MSAWhlTqReq_Nm]
  VINP_CrashSignalGPIO_flg/1 -> [VINP_CrashSignalGPIO_flg]
  VINP_CrashOutputSts_enum/1 -> [VINP_CrashOutputSts_enum]
  [VPMM_PowerSta_enum] -> CrashDetect/1(VPMM_PowerSta_enum)
  [VINP_CrashSignalGPIO_flg] -> CrashDetect/2(VINP_CrashSignalGPIO_flg)
  [VINP_CrashOutputSts_enum] -> CrashDetect/3(VINP_CrashOutputSts_enum)
  [task_time_s] -> CrashDetect/4(task_time_s)
  CrashDetect/1(VTQD_CrashDetd_flg) -> VTQD_CrashDetd_flg/1  "VTQD_CrashDetd_flg"
  CrashDetect/2(VTQD_DiagHCrash_flg) -> VTQD_DiagHCrash_flg/1  "VTQD_DiagHCrash_flg"
  VINP_LongAccel_Gps/1 -> [VINP_LongAccel_Gps]
  [VINP_LongAccel_Gps] -> TorqueModule/48(VINP_LongAccel_Gps)
  TorqueModule/44(VTQD_ReBrakeLPReq_flg) -> VTQD_ReBrakeLPReq_flg/1
  VTQR_ActualFEDUWhlTqReq_Nm/1 -> [VTQR_ActualFEDUWhlTqReq_Nm]
  VTQR_ActualREDUWhlTqReq_Nm/1 -> [VTQR_ActualREDUWhlTqReq_Nm]
  [VTQR_ActualFEDUWhlTqReq_Nm] -> TorqueModule/49(VTQR_ActualFEDUWhlTqReq_Nm)
  [VTQR_ActualREDUWhlTqReq_Nm] -> TorqueModule/50(VTQR_ActualREDUWhlTqReq_Nm)
  [VINP_BrkPedalPos_pct] -> TorqueModule/51(VINP_BrkPedalPos_pct)
  [VTQD_RDCActive_enum] -> TorqueModule/52(VTQD_RDCActive_enum)
  VINP_EPBCarWashMode_flg/1 -> [VINP_EPBCarWashMode_flg]
  VINP_EPBErrSta_enum/1 -> [VINP_EPBErrSta_enum]
  VINP_EPBSta_enum/1 -> [VINP_EPBSta_enum]
  VINP_DOASta_flg/1 -> [VINP_DOASta_flg]
  VINP_FrMotorAvailTq_Nm/1 -> [VINP_FrMotorAvailTq_Nm]
  VINP_RrMotorAvailTq_Nm/1 -> [VINP_RrMotorAvailTq_Nm]
  [VINP_FrMotorAvailTq_Nm] -> TorqueModule/54(VINP_FrMotorAvailTq_Nm)
  [VINP_RrMotorAvailTq_Nm] -> TorqueModule/55(VINP_RrMotorAvailTq_Nm)
  [task_time_s] -> TorqueModule/56(task_time_s)
  TorqueModule/45(VTQD_LoSpdBrkCtrl_flg) -> VTQD_LoSpdBrkCtrl_flg/1
  TorqueModule/46(VTQD_BOSEnable_flg) -> VTQD_BOSEnable_flg/1
  TorqueModule/52(VTQD_APSStaSys_enum) -> VTQD_APSStaSys_enum/1
  TorqueModule/53(VTQD_APSReq_enum) -> VTQD_APSReq_enum/1
  TorqueModule/54(VTQD_APSDecReqA_flg) -> VTQD_APSDecReqA_flg/1
  TorqueModule/55(VTQD_APSDecReq_mps2) -> VTQD_APSDecReq_mps2/1
  VINP_HSAActive_flg/1 -> [VINP_HSAActive_flg]
  VTQR_NoABSREDUWhlTqReq_Nm/1 -> [VTQR_NoABSREDUWhlTqReq_Nm]
  VTQR_NoABSFEDUWhlTqReq_Nm/1 -> [VTQR_NoABSFEDUWhlTqReq_Nm]
  VINP_GRADE_Deg/1 -> [VINP_GRADE_Deg]
  VINP_AVHActive_flg/1 -> [VINP_AVHActive_flg]
  VINP_DrDoorSW_flg/1 -> [VINP_DrDoorSW_flg]
  VINP_MCUWarnF_enum/1 -> [VINP_MCUWarnF_enum]
  VINP_MCUWarnR_enum/1 -> [VINP_MCUWarnR_enum]
  VVMC_APSSpeedCMD_kph/1 -> [VVMC_APSSpeedCMD_kph]
  VVMC_APSShiftPosnReq_enum/1 -> [VVMC_APSShiftPosnReq_enum]
  VINP_DriverSeatBeltCmd_flg/1 -> [VINP_DriverSeatBeltCmd_flg]
  VINP_ChrgPlugSta_enum/1 -> [VINP_ChrgPlugSta_enum]
  VINP_SeatSW_flg/1 -> [VINP_SeatSW_flg]
  [VINP_MCUWarnF_enum] -> Signal_convert/17(VINP_MCUWarnF_enum)
  [task_time_s] -> Signal_convert/19(task_time_s)
  [VINP_FrEDURealTMTq_Nm] -> Signal_convert/20(VINP_FrEDURealTMTq_Nm)
  [VINP_RrEDURealTMTq_Nm] -> Signal_convert/21(VINP_RrEDURealTMTq_Nm)
  [VINP_GRADE_Deg] -> Signal_convert/22(VINP_GRADE_Deg)
  [VINP_MCUWarnR_enum] -> Signal_convert/18(VINP_MCUWarnR_enum)
  [VINP_HSAActive_flg] -> TorqueModule/57(VINP_HSAActive_flg)
  [VTQR_NoABSFEDUWhlTqReq_Nm] -> TorqueModule/58(VTQR_NoABSFEDUWhlTqReq_Nm)
  [VTQR_NoABSREDUWhlTqReq_Nm] -> TorqueModule/59(VTQR_NoABSREDUWhlTqReq_Nm)
  [VINP_AVHActive_flg] -> TorqueModule/60(VINP_AVHActive_flg)
  [VINP_EPBErrSta_enum] -> TorqueModule/61(VINP_EPBErrSta_enum)
  Signal_convert/17(VTQD_EstVehWeightResult_kg) -> [VTQD_EstVehWeightResult_kg]
  [VTQD_EPBCarWashMode_flg] -> ShiftModule/8(VTQD_EPBCarWashMode_flg)
  [VINP_DrDoorSW_flg] -> ShiftModule/9(VINP_DrDoorSW_flg)
  [VVMC_APSShiftPosnReq_enum] -> ShiftModule/10(VVMC_APSShiftPosnReq_enum)
  [VVMC_APSActive_flg] -> ShiftModule/11(VVMC_APSActive_flg)
  [VINP_DriverSeatBeltCmd_flg] -> ShiftModule/12(VINP_DriverSeatBeltCmd_flg)
  [VINP_SeatSW_flg] -> ShiftModule/13(VINP_SeatSW_flg)
  [VINP_ChrgPlugSta_enum] -> ShiftModule/14(VINP_ChrgPlugSta_enum)
  [VTQD_IVIPwrLock_flg] -> ShiftModule/15(VTQD_IVIPwrLock_flg)
  VINP_IVICreepSWReq_flg/1 -> [VINP_IVICreepSWReq_flg]
  TorqueModule/47(VTQD_ExtShftAllow_flg) -> VTQD_ExtShftAllow_flg/1
  TorqueModule/19(VTQD_FrEDUActTqValid_flg) -> Terminator/1
  TorqueModule/20(VTQD_FrEDURolRgnTqValid_flg) -> Terminator1/1
  [VINP_IVICreepSWReq_flg] -> Signal_convert/23(VINP_IVICreepSWReq_flg)
  VPMM_SysPowerMode_enum/1 -> [VPMM_SysPowerMode_enum]
  [VPMM_SysPowerMode_enum] -> Signal_convert/24(VPMM_SysPowerMode_enum)
  TorqueModule/48(VTQD_OPDOn2Off_flg) -> [VTQD_OPDOn2Off_flg]
  [VTQD_OPDOn2Off_flg] -> Signal_convert/26(VTQD_OPDOn2Off_flg)
  [VTQD_AfterAvailableTqDemFr_Nm] -> ShiftModule/16(VTQD_AfterAvailableTqDemFr_Nm)
  [VTQD_AfterAvailableTqDemRr_Nm] -> ShiftModule/17(VTQD_AfterAvailableTqDemRr_Nm)
  [VTQR_NoABSREDUWhlTqReq_Nm] -> ShiftModule/19(VTQR_NoABSREDUWhlTqReq_Nm)
  [VTQR_NoABSFEDUWhlTqReq_Nm] -> ShiftModule/18(VTQR_NoABSFEDUWhlTqReq_Nm)
  TorqueModule/49(VTQD_PreLoadHold_flg) -> VTQD_PreLoadHold_flg/1
  TorqueModule/50(VTQD_PreLoadPreEn_flg) -> VTQD_PreLoadPreEn_flg/1
  [VINP_DOASta_flg] -> ShiftModule/20(VINP_DOASta_flg)
  VVMC_ACCRequiredAccel_mps2/1 -> [VVMC_ACCRequiredAccel_mps2]
  [VINP_FrntAxlTrqReqBrk_Nm] -> Signal_convert/27(VINP_FrntAxlTrqReqBrk_Nm)
  [VINP_RearAxlTrqReqBrk_Nm] -> Signal_convert/28(VINP_RearAxlTrqReqBrk_Nm)
  [VINP_FrRBCActive_flg] -> Signal_convert/29(VINP_FrRBCActive_flg)
  [VINP_RrRBCActive_flg] -> Signal_convert/30(VINP_RrRBCActive_flg)
  [VVMC_ADASActive_flg] -> Signal_convert/31(VVMC_ADASActive_flg)
  [VVMC_ACCRequiredAccel_mps2] -> Signal_convert/32(VVMC_ACCRequiredAccel_mps2)
  TorqueModule/51(VTQD_CreepPrLoadEnable_flg) -> VTQD_CreepPrLoadEnable_flg/1
  Signal_convert/18(VTQD_RDCActive_enum) -> [VTQD_RDCActive_enum]
  VINP_ACCVehHoldReq_flg/1 -> [VINP_ACCVehHoldReq_flg]
  [VINP_ACCVehHoldReq_flg] -> TorqueModule/64(VINP_ACCVehHoldReq_flg)
  VVMC_ACCPedalOvrd_flg/1 -> [VVMC_ACCPedalOvrd_flg]
  [VVMC_ACCPedalOvrd_flg] -> Signal_convert/33(VVMC_ACCPedalOvrd_flg)
  ShiftModule/6(VTQD_DriveProtRemove_flg) -> [VTQD_DriveProtRemove_flg]
  [VTQD_DriveProtRemove_flg] -> TorqueModule/65(VTQD_DriveProtRemove_flg)
  [VTQD_AfterAvailableTqDemFr_Nm] -> Signal_convert/34(VTQD_AfterAvailableTqDemFr_Nm)
  [VTQD_AfterAvailableTqDemRr_Nm] -> Signal_convert/35(VTQD_AfterAvailableTqDemRr_Nm)
  ShiftModule/7(VTQD_DriveProtEn_flg) -> VTQD_DriveProtEn_flg/1
  [VVMC_ACCRequiredAccel_mps2] -> TorqueModule/66(VVMC_ACCRequiredAccel_mps2)
  [VVMC_ADASWhlTqReq_Nm] -> Signal_convert/36(VVMC_ADASWhlTqReq_Nm)
  [VTQR_NoABSREDUWhlTqReq_Nm] -> Signal_convert/37(VTQR_NoABSREDUWhlTqReq_Nm)
  [VTQR_NoABSFEDUWhlTqReq_Nm] -> Signal_convert/38(VTQR_NoABSFEDUWhlTqReq_Nm)
  Signal_convert/20(VTQD_EPBCarWashMode_flg) -> [VTQD_EPBCarWashMode_flg]
  [VTQD_EstVehWeightResult_kg] -> TorqueModule/32(VTQD_EstVehWeightResult_kg)
  [VVMC_LongAcc_Gps] -> TorqueModule/33(VVMC_LongAcc_Gps)
  TorqueModule/56(VTQD_ActParkRequest_flg) -> VTQD_ActParkRequest_flg/1
  VINP_PsngrSeatBeltCmd_flg/1 -> [VINP_PsngrSeatBeltCmd_flg]
  VINP_RDriverSeatBeltCmd_flg/1 -> [VINP_RDriverSeatBeltCmd_flg]
  VINP_RCenterSeatBeltCmd_flg/1 -> [VINP_RCenterSeatBeltCmd_flg]
  VINP_RPsngrSeatBeltCmd_flg/1 -> [VINP_RPsngrSeatBeltCmd_flg]
  VINP_RollModeSWCmd_enum/1 -> [VINP_RollModeSWCmd_enum]
  VVMC_LongAcc_Gps/1 -> [VVMC_LongAcc_Gps]
  VVMC_ActMaxSlideRate_pct/1 -> [VVMC_ActMaxSlideRate_pct]
  [VVMC_LongAcc_Gps] -> Signal_convert/39(VVMC_LongAcc_Gps)
  [VINP_DOASta_flg] -> Signal_convert/47(VINP_DOASta_flg)
  [VINP_EPBCarWashMode_flg] -> Signal_convert/46(VINP_EPBCarWashMode_flg)
  [VINP_RollModeSWCmd_enum] -> Signal_convert/45(VINP_RollModeSWCmd_enum)
  [VINP_RPsngrSeatBeltCmd_flg] -> Signal_convert/44(VINP_RPsngrSeatBeltCmd_flg)
  [VINP_RCenterSeatBeltCmd_flg] -> Signal_convert/43(VINP_RCenterSeatBeltCmd_flg)
  [VINP_RDriverSeatBeltCmd_flg] -> Signal_convert/42(VINP_RDriverSeatBeltCmd_flg)
  [VINP_PsngrSeatBeltCmd_flg] -> Signal_convert/41(VINP_PsngrSeatBeltCmd_flg)
  [VINP_DriverSeatBeltCmd_flg] -> Signal_convert/40(VINP_DriverSeatBeltCmd_flg)
  [VVMC_APSSpeedCMD_kph] -> TorqueModule/62(VVMC_APSSpeedCMD_kph)
  [VVMC_ActMaxSlideRate_pct] -> TorqueModule/53(VVMC_ActMaxSlideRate_pct)
  VVMC_EstSlope_Deg/1 -> [VVMC_EstSlope_Deg]
  [VVMC_EstSlope_Deg] -> TorqueModule/67(VVMC_EstSlope_Deg)
  TorqueModule/57(VTQD_RegenTqLimitEn_flg) -> VTQD_RegenTqLimitEn_flg/1
  [VINP_IVIPwrLockSW_enum] -> Signal_convert/49(VINP_IVIPwrLockSW_enum)
  [VVMC_RWDRDCActive_enum] -> Signal_convert/48(VVMC_RWDRDCActive_enum)
  Signal_convert/21(VTQD_IVIPwrLock_flg) -> [VTQD_IVIPwrLock_flg]
  [VTQD_SysMode_enum] -> TorqueModule/68(VTQD_SysMode_enum)
  [VINP_SWCResUpSta_flg] -> TorqueModule/69(VINP_SWCResUpSta_flg)
  [VINP_DrDoorSW_flg] -> TorqueModule/70(VINP_DrDoorSW_flg)
  [VINP_PsDoorSW_flg] -> TorqueModule/71(VINP_PsDoorSW_flg)
  [VINP_RRDoorSW_flg] -> TorqueModule/72(VINP_RRDoorSW_flg)
  [VINP_RLDoorSW_flg] -> TorqueModule/73(VINP_RLDoorSW_flg)
  [VINP_HoodSW_flg] -> TorqueModule/74(VINP_HoodSW_flg)
  [VINP_TailgateSW_flg] -> TorqueModule/75(VINP_TailgateSW_flg)
  [VINP_ADASACCSta_enum] -> TorqueModule/76(VINP_ADASACCSta_enum)
  [VINP_EPBSta_enum] -> TorqueModule/77(VINP_EPBSta_enum)
  TorqueModule/58(VTQD_ExtDoorAllow_flg) -> VTQD_ExtDoorAllow_flg/1
  VINP_RLDoorSW_flg/1 -> [VINP_RLDoorSW_flg]
  VINP_HoodSW_flg/1 -> [VINP_HoodSW_flg]
  VINP_PsDoorSW_flg/1 -> [VINP_PsDoorSW_flg]
  VINP_TailgateSW_flg/1 -> [VINP_TailgateSW_flg]
  VINP_RRDoorSW_flg/1 -> [VINP_RRDoorSW_flg]
  VINP_IVIPwrLockSW_enum/1 -> [VINP_IVIPwrLockSW_enum]
  VVMC_RWDRDCActive_enum/1 -> [VVMC_RWDRDCActive_enum]
  VVMC_APSReq_enum/1 -> [VVMC_APSReq_enum]
  [VVMC_APSReq_enum] -> TorqueModule/63(VVMC_APSReq_enum)
  VINP_SWCResUpSta_flg/1 -> [VINP_SWCResUpSta_flg]
  [VVMC_ActRRSlideRate_pct] -> TorqueModule/79(VVMC_ActRRSlideRate_pct)
  [VVMC_ActLRSlideRate_pct] -> TorqueModule/78(VVMC_ActLRSlideRate_pct)
  VVMC_ActRRSlideRate_pct/1 -> [VVMC_ActRRSlideRate_pct]
  VVMC_ActLRSlideRate_pct/1 -> [VVMC_ActLRSlideRate_pct]
  [VVMC_ActStESCYaw_degps] -> TorqueModule/82(VVMC_ActStESCYaw_degps)
  [VINP_YawRate_degps] -> TorqueModule/81(VINP_YawRate_degps)
  [VINP_SASAngle_Deg] -> TorqueModule/80(VINP_SASAngle_Deg)
  VINP_SASAngle_Deg/1 -> [VINP_SASAngle_Deg]
  VINP_YawRate_degps/1 -> Switch/3
  VVMC_ActStESCYaw_degps/1 -> [VVMC_ActStESCYaw_degps]
  TorqueModule/6(VTQD_AfterAvailableTqDemFr_Nm) -> [VTQD_AfterAvailableTqDemFr_Nm], VTQD_AfterAvailableTqDemFr_Nm/1
  [VVMC_CAASActive_flg] -> TorqueModule/83(VVMC_CAASActive_flg)
  TorqueModule/59(VTQD_WhlTqCapGenFr_Nm) -> VTQD_WhlTqCapGenFr_Nm/1, [VTQD_WhlTqCapGenFr_Nm]
  TorqueModule/60(VTQD_WhlTqCapGenRr_Nm) -> VTQD_WhlTqCapGenRr_Nm/1, [VTQD_WhlTqCapGenRr_Nm]
  [VINP_HVBattSOC_pct] -> TorqueModule/84(VINP_HVBattSOC_pct)
  VINP_HVBattSOC_pct/1 -> [VINP_HVBattSOC_pct]
  Signal_convert/23(VTQD_RegenMode_enum) -> [VTQD_RegenMode_enum]
  TorqueModule/61(VTQD_OPDHoldAllowPark_flg) -> [VTQD_OPDHoldAllowPark_flg]
  [VTQD_OPDHoldAllowPark_flg] -> ShiftModule/21(VTQD_OPDHoldAllowPark_flg)
  TorqueModule/62(VTQD_OPDHoldLamp_flg) -> VTQD_OPDHoldLamp_flg/1
  [VTQD_LowIdleAccPedal_flg] -> VTQD_LowIdleAccPedal_flg/1
  [VTQD_CreepON_flg] -> VTQD_CreepON_flg/1
  [VTQD_EstVehWeightResult_kg] -> VTQD_EstVehWeightResult_kg/1
  [VTQD_RDCActive_enum] -> VTQD_RDCActive_enum/1
  [VTQD_RegenMode_enum] -> VTQD_RegenMode_enum/1
  [VTQD_EquivAccPedalSWSta_flg] -> VTQD_EquivAccPedalSWSta_flg/1
  Signal_convert/19(VTQD_EquivAccPedalSWSta_flg) -> [VTQD_EquivAccPedalSWSta_flg]
  [VTQD_IVIPwrLockSta_enum] -> VTQD_IVIPwrLockSta_enum/1
  Signal_convert/22(VTQD_IVIPwrLockSta_enum) -> [VTQD_IVIPwrLockSta_enum]
  [VPMM_PowerSta_enum] -> Signal_convert/25(VPMM_PowerSta_enum)
  [VINP_ADASACCSta_enum] -> Signal_convert/50(VINP_ADASACCSta_enum)
  VINP_ADASACCSta_enum/1 -> [VINP_ADASACCSta_enum]
  [VVMC_CCCtrlSta_enum] -> Signal_convert/51(VVMC_CCCtrlSta_enum)
  [VINP_ADASISASta_enum] -> Signal_convert/52(VINP_ADASISASta_enum)
  [VINP_IVIISAOffsetSpd_enum] -> Signal_convert/53(VINP_IVIISAOffsetSpd_enum)
  [VVMC_MSACtrlSta_enum] -> Signal_convert/54(VVMC_MSACtrlSta_enum)
  [VINP_ADASVehSpdLim_kph] -> Signal_convert/55(VINP_ADASVehSpdLim_kph)
  [VBCM_BrakeLamp_flg] -> Signal_convert/56(VBCM_BrakeLamp_flg)
  VINP_ADASVehSpdLim_kph/1 -> [VINP_ADASVehSpdLim_kph]
  VVMC_CAASActive_flg/1 -> [VVMC_CAASActive_flg]
  VVMC_MSACtrlSta_enum/1 -> [VVMC_MSACtrlSta_enum]
  VVMC_CCCtrlSta_enum/1 -> [VVMC_CCCtrlSta_enum]
  VINP_ADASISASta_enum/1 -> [VINP_ADASISASta_enum]
  VINP_IVIISAOffsetSpd_enum/1 -> [VINP_IVIISAOffsetSpd_enum]
  VBCM_BrakeLamp_flg/1 -> [VBCM_BrakeLamp_flg]
  [VINP_SWCResUpSta_flg] -> Signal_convert/57(VINP_SWCResUpSta_flg)
  [VINP_SWCSetdownSta_flg] -> Signal_convert/58(VINP_SWCSetdownSta_flg)
  [VINP_SWCACCSta_flg] -> Signal_convert/59(VINP_SWCACCSta_flg)
  [VINP_SWCCANCELSta_flg] -> Signal_convert/60(VINP_SWCCANCELSta_flg)
  [VINP_SWCRegenUp_flg] -> Signal_convert/61(VINP_SWCRegenUp_flg)
  [VINP_SWCRegenDown_flg] -> Signal_convert/62(VINP_SWCRegenDown_flg)
  VINP_SWCSetdownSta_flg/1 -> [VINP_SWCSetdownSta_flg]
  VINP_SWCACCSta_flg/1 -> [VINP_SWCACCSta_flg]
  VINP_SWCCANCELSta_flg/1 -> [VINP_SWCCANCELSta_flg]
  VINP_SWCRegenUp_flg/1 -> [VINP_SWCRegenUp_flg]
  VINP_SWCRegenDown_flg/1 -> [VINP_SWCRegenDown_flg]
  Signal_convert/28(VTQD_SetSpd_kph) -> [VTQD_SetSpd_kph]
  Signal_convert/24(VTQD_SaveRegenMode_enum) -> [VTQD_SaveRegenMode_enum]
  Signal_convert/25(VTQD_FDCVCURegenMode_enum) -> [VTQD_FDCVCURegenMode_enum]
  Signal_convert/26(VTQD_SpdCtrlMode_enum) -> [VTQD_SpdCtrlMode_enum]
  Signal_convert/27(VTQD_SpdCtrlSta_flg) -> [VTQD_SpdCtrlSta_flg]
  [VTQD_SaveRegenMode_enum] -> VTQD_SaveRegenMode_enum/1
  [VTQD_FDCVCURegenMode_enum] -> VTQD_FDCVCURegenMode_enum/1
  [VTQD_SpdCtrlMode_enum] -> VTQD_SpdCtrlMode_enum/1
  [VTQD_SpdCtrlSta_flg] -> VTQD_SpdCtrlSta_flg/1
  [VTQD_SetSpd_kph] -> VTQD_SetSpd_kph/1
  VINP_FlashRegenMode_enum/1 -> [VINP_FlashRegenMode_enum]
  [VINP_FlashRegenMode_enum] -> Signal_convert/63(VINP_FlashRegenMode_enum)
  Signal_convert/31(VTQD_SWCCancelSta_flg) -> VTQD_SWCCancelSta_flg/1  "VTQD_SWCCancelSta_flg"
  Signal_convert/30(VTQD_SWCSetdownSta_flg) -> VTQD_SWCSetdownSta_flg/1  "VTQD_SWCSetdownSta_flg"
  Signal_convert/29(VTQD_SWCResUpSta_flg) -> VTQD_SWCResUpSta_flg/1  "VTQD_SWCResUpSta_flg"
  TorqueModule/63(VTQD_CreepBaseTqD_Nm) -> VTQD_CreepBaseTqD_Nm/1
  Switch/1 -> [VINP_YawRate_degps]  "VINP_YawRate_degps"
  Constant21/1 -> Switch/2
  VVMC_CalibratedGyroY_Dps/1 -> Switch/1
  TorqueModule/64(VTQD_VehActSpd_kph) -> VTQD_VehActSpd_kph/1, [VTQD_VehActSpd_kph]
  [VINP_HVBattSOCDis_pct] -> Signal_convert/68(VINP_HVBattSOCDis_pct)
  [VINP_HVBMTempMax_C] -> Signal_convert/69(VINP_HVBMTempMax_C)
  [VINP_HVBMTempMin_C] -> Signal_convert/70(VINP_HVBMTempMin_C)
  Signal_convert/32(VTQD_RegenLimIndSta_flg) -> VTQD_RegenLimIndSta_flg/1
  VINP_HVBMTempMin_C/1 -> [VINP_HVBMTempMin_C]
  VINP_HVBattSOCDis_pct/1 -> [VINP_HVBattSOCDis_pct]
  VINP_HVBMTempMax_C/1 -> [VINP_HVBMTempMax_C]
  [VINP_SmartEcoModeSW_flg] -> Signal_convert/71(VINP_SmartEcoModeSW_flg)
  VINP_SmartEcoModeSW_flg/1 -> [VINP_SmartEcoModeSW_flg]
  TorqueModule/65(VTQD_CoordTqDem_Nm) -> [VTQD_CoordTqDem_Nm]
  [VTQD_CoordTqDem_Nm] -> Signal_convert/72(VTQD_CoordTqDem_Nm)
  [VINP_ESCActive_flg] -> TorqueModule/86(VINP_ESCActive_flg)
  [VINP_ABSActive_flg] -> TorqueModule/87(VINP_ABSActive_flg)
  VINP_ESCActive_flg/1 -> [VINP_ESCActive_flg]
  VINP_ABSActive_flg/1 -> [VINP_ABSActive_flg]
  VINP_CAASSta_enum/1 -> [VINP_CAASSta_enum]
  [VINP_CAASSta_enum] -> ShiftModule/22(VAPM_CAASSta_enum)
  VVMC_SetACCDisableAPS_flg/1 -> [VVMC_SetACCDisableAPS_flg]
  [VVMC_SetACCDisableAPS_flg] -> Signal_convert/73(VVMC_SetACCDisableAPS_flg)
  [VINP_IVISnowModeCmd_flg] -> TorqueModule/88(VINP_IVISnowModeCmd_flg)
  [VINP_IVISnowModeCmd_flg] -> Signal_convert/74(VINP_IVISnowModeCmd_flg)
  [VINP_SWC2LScrollUpSta_flg] -> Signal_convert/75(VINP_SWC2LScrollUpSta_flg)
  [VINP_SWC2LScrollDownSta_flg] -> Signal_convert/76(VINP_SWC2LScrollDownSta_flg)
  [VINP_SWC2LScrollPressSta_flg] -> Signal_convert/77(VINP_SWC2LScrollPressSta_flg)
  [VINP_SWC2LADASSta_flg] -> Signal_convert/78(VINP_SWC2LADASSta_flg)
  [VVMC_MSAActive_flg] -> Signal_convert/79(VVMC_MSAActive_flg)
  [VINP_ADASSLIFSpdLim_enum] -> Signal_convert/80(VINP_ADASSLIFSpdLim_enum)
  [VINP_IVIACCAdaptiveSta_flg] -> Signal_convert/81(VINP_IVIACCAdaptiveSta_flg)
  Signal_convert/38(VTQD_SetSpdLimWarn_flg) -> VTQD_SetSpdLimWarn_flg/1
  Signal_convert/33(VTQD_SWC2CancelSta_flg) -> VTQD_SWC2CancelSta_flg/1
  Signal_convert/34(VTQD_SWC2SetdownSta_flg) -> VTQD_SWC2SetdownSta_flg/1
  Signal_convert/35(VTQD_SWC2ResUpSta_flg) -> VTQD_SWC2ResUpSta_flg/1
  Signal_convert/36(VTQD_SWC2LADASSta_flg) -> VTQD_SWC2LADASSta_flg/1
  Signal_convert/37(VTQD_SpdLim4SetSpd_raw32) -> VTQD_SpdLim4SetSpd_raw32/1
  VINP_ADASSLIFSpdLim_enum/1 -> [VINP_ADASSLIFSpdLim_enum]
  VINP_SWC2LADASSta_flg/1 -> [VINP_SWC2LADASSta_flg]
  VINP_IVISnowModeCmd_flg/1 -> [VINP_IVISnowModeCmd_flg]
  VINP_SWC2LScrollUpSta_flg/1 -> [VINP_SWC2LScrollUpSta_flg]
  VINP_SWC2LScrollDownSta_flg/1 -> [VINP_SWC2LScrollDownSta_flg]
  VINP_SWC2LScrollPressSta_flg/1 -> [VINP_SWC2LScrollPressSta_flg]
  [VINP_VehicleType_enum] -> TorqueModule/89(VINP_VehicleType_enum)
  VINP_VehicleType_enum/1 -> [VINP_VehicleType_enum]
  VINP_IVIACCAdaptiveSta_flg/1 -> [VINP_IVIACCAdaptiveSta_flg]
  [VINP_SWCType_enum] -> Signal_convert/82(VINP_SWCType_enum)
  VINP_SWCType_enum/1 -> [VINP_SWCType_enum]
  VINP_Distanceunit_flg/1 -> [VINP_Distanceunit_flg]
  VVMC_MeterIndSpeed_raw32/1 -> [VVMC_MeterIndSpeed_raw32]
  VVMC_ACCObjDist_m/1 -> [VVMC_ACCObjDist_m]
  VVMC_LVDAACCStatusInformation_flg/1 -> [VVMC_LVDAACCStatusInformation_flg]
  [VINP_Distanceunit_flg] -> Signal_convert/67(VINP_Distanceunit_flg)
  [VVMC_MeterIndSpeed_raw32] -> Signal_convert/66(VVMC_MeterIndSpeed_raw32)
  [VVMC_ACCObjDist_m] -> Signal_convert/65(VVMC_ACCObjDist_m)
  [VVMC_LVDAACCStatusInformation_flg] -> Signal_convert/64(VVMC_LVDAACCStatusInformation_flg)
  [VVMC_RearTqRatio_rat] -> TorqueModule/85(VVMC_RearTqRatio_rat)
  VVMC_RearTqRatio_rat/1 -> [VVMC_RearTqRatio_rat]
  [VINP_RRRawWhlSpeed_kph] -> Signal_convert/86(VINP_RRRawWhlSpeed_kph)
  [VINP_RFRawWhlSpeed_kph] -> Signal_convert/85(VINP_RFRawWhlSpeed_kph)
  [VINP_LRRawWhlSpeed_kph] -> Signal_convert/84(VINP_LRRawWhlSpeed_kph)
  [VINP_LFRawWhlSpeed_kph] -> Signal_convert/83(VINP_LFRawWhlSpeed_kph)
  VINP_RRRawWhlSpeed_kph/1 -> [VINP_RRRawWhlSpeed_kph]
  VINP_LFRawWhlSpeed_kph/1 -> [VINP_LFRawWhlSpeed_kph]
  VINP_LRRawWhlSpeed_kph/1 -> [VINP_LRRawWhlSpeed_kph]
  VINP_RFRawWhlSpeed_kph/1 -> [VINP_RFRawWhlSpeed_kph]
  [VINP_IVITrailerModeSWSta_flg] -> Signal_convert/87(VINP_IVITrailerModeSWSta_flg)
  [VBCM_UserNow_enum] -> Signal_convert/88(VBCM_UserNow_enum)
  [VBCM_RegenModeUserSetting_enum] -> Signal_convert/89(VBCM_RegenModeUserSetting_enum)
  VBCM_UserNow_enum/1 -> [VBCM_UserNow_enum]
  VINP_IVITrailerModeSWSta_flg/1 -> [VINP_IVITrailerModeSWSta_flg]
  VBCM_RegenModeUserSetting_enum/1 -> [VBCM_RegenModeUserSetting_enum]
  [VINP_SWC2RScrollPressSta_flg] -> Signal_convert/90(VINP_SWC2RScrollPressSta_flg)
  [VINP_SWC2RScrollUpSta_flg] -> Signal_convert/91(VINP_SWC2RScrollUpSta_flg)
  [VINP_SWC2RScrollDownSta_flg] -> Signal_convert/92(VINP_SWC2RScrollDownSta_flg)
  [VINP_SWC2LDriveModeSta_flg] -> Signal_convert/93(VINP_SWC2LDriveModeSta_flg)
  [VINP_SWC2RRightSta_flg] -> Signal_convert/94(VINP_SWC2RRightSta_flg)
  [VINP_SWC2RLeftSta_flg] -> Signal_convert/95(VINP_SWC2RLeftSta_flg)
  VINP_SWC2RLeftSta_flg/1 -> [VINP_SWC2RLeftSta_flg]
  VINP_SWC2LDriveModeSta_flg/1 -> [VINP_SWC2LDriveModeSta_flg]
  VINP_SWC2RScrollDownSta_flg/1 -> [VINP_SWC2RScrollDownSta_flg]
  VINP_SWC2RRightSta_flg/1 -> [VINP_SWC2RRightSta_flg]
  VINP_SWC2RScrollUpSta_flg/1 -> [VINP_SWC2RScrollUpSta_flg]
  VINP_SWC2RScrollPressSta_flg/1 -> [VINP_SWC2RScrollPressSta_flg]
  Signal_convert/39(VTQD_MaxWhlSlideRate_pct) -> VTQD_MaxWhlSlideRate_pct/1
  Signal_convert/40(VTQD_MinWhlSlideRate_pct) -> VTQD_MinWhlSlideRate_pct/1
  Signal_convert/41(VTQD_LeftSlideRate_pct) -> VTQD_LeftSlideRate_pct/1
  Signal_convert/42(VTQD_RightSlideRate_pct) -> VTQD_RightSlideRate_pct/1
  Signal_convert/43(VTQD_FrontSlideRate_pct) -> [VTQD_FrontSlideRate_pct], VTQD_FrontSlideRate_pct/1
  Signal_convert/44(VTQD_RearSlideRate_pct) -> [VTQD_RearSlideRate_pct], VTQD_RearSlideRate_pct/1
  Signal_convert/45(VTQD_TrailerDisOPDSta_flg) -> VTQD_TrailerDisOPDSta_flg/1
  Signal_convert/46(VTQD_ComboKeyPreEn_flg) -> VTQD_ComboKeyPreEn_flg/1
  Signal_convert/47(VTQD_ComboKeyEn_flg) -> VTQD_ComboKeyEn_flg/1
  Signal_convert/48(VTQD_SysMode_enum) -> [VTQD_SysMode_enum], VTQD_SysMode_enum/1
  VINP_IVIEscapeModeCmd_flg/1 -> [VINP_IVIEscapeModeCmd_flg]
  [VTQD_IVIRockModeEn_flg] -> ShiftModule/23(VTQD_IVIRockModeEn_flg)
  [VTQD_IVIRockModeEn_flg] -> TorqueModule/90(VTQD_IVIRockModeEn_flg)
  [VTQR_RShaftSpdTqLimLow_flg] -> TorqueModule/91(VTQR_RShaftSpdTqLimLow_flg)
  [VTQR_RTimerTqLimLow_flg] -> TorqueModule/92(VTQR_RTimerTqLimLow_flg)
  [VTQR_FShaftSpdTqLimLow_flg] -> TorqueModule/93(VTQR_FShaftSpdTqLimLow_flg)
  [VTQR_FTimerTqLimLow_flg] -> TorqueModule/94(VTQR_FTimerTqLimLow_flg)
  [VINP_LFRawWhlSpeed_kph] -> TorqueModule/95(VINP_LFRawWhlSpeed_kph)
  [VINP_LRRawWhlSpeed_kph] -> TorqueModule/96(VINP_LRRawWhlSpeed_kph)
  [VINP_RFRawWhlSpeed_kph] -> TorqueModule/97(VINP_RFRawWhlSpeed_kph)
  [VINP_RRRawWhlSpeed_kph] -> TorqueModule/98(VINP_RRRawWhlSpeed_kph)
  VTQR_RTimerTqLimLow_flg/1 -> [VTQR_RTimerTqLimLow_flg]
  VTQR_RShaftSpdTqLimLow_flg/1 -> [VTQR_RShaftSpdTqLimLow_flg]
  VTQR_FShaftSpdTqLimLow_flg/1 -> [VTQR_FShaftSpdTqLimLow_flg]
  VTQR_FTimerTqLimLow_flg/1 -> [VTQR_FTimerTqLimLow_flg]
  [VTQD_RearSlideRate_pct] -> TorqueModule/99(VTQD_RearSlideRate_pct)
  [VTQD_FrontSlideRate_pct] -> TorqueModule/100(VTQD_FrontSlideRate_pct)
  TorqueModule/66(VTQD_PedAccTqEn_flg) -> VTQD_PedAccTqEn_flg/1
  TorqueModule/67(VTQD_WhlTqCapMotFr_Nm) -> VTQD_WhlTqCapMotFr_Nm/1
  TorqueModule/68(VTQD_WhlTqCapMotRr_Nm) -> VTQD_WhlTqCapMotRr_Nm/1
  VINP_SWC2RCustomizeSta_flg/1 -> [VINP_SWC2RCustomizeSta_flg]
  [VINP_SWC2RCustomizeSta_flg] -> TorqueModule/101(VINP_SWC2RCustomizeSta_flg)
  [VTQD_VehActSpd_kph] -> Signal_convert/96(VTQD_VehActSpd_kph)
  VTQR_FrFirstOrderInpTs_c/1 -> [VTQR_FrFirstOrderInpTs_c]
  VTQR_FrRateLimitInc_Nm/1 -> [VTQR_FrRateLimitInc_Nm]
  VTQR_FrRateLimitDec_Nm/1 -> [VTQR_FrRateLimitDec_Nm]
  VTQR_RrFirstOrderInpTs_c/1 -> [VTQR_RrFirstOrderInpTs_c]
  VTQR_RrRateLimitDec_Nm/1 -> [VTQR_RrRateLimitDec_Nm]
  VTQR_RrRateLimitInc_Nm/1 -> [VTQR_RrRateLimitInc_Nm]
  [VTQR_FrFirstOrderInpTs_c] -> TorqueModule/102(VTQR_FrFirstOrderInpTs_c)
  [VTQR_RrFirstOrderInpTs_c] -> TorqueModule/103(VTQR_RrFirstOrderInpTs_c)
  [VTQR_FrRateLimitInc_Nm] -> TorqueModule/104(VTQR_FrRateLimitInc_Nm)
  [VTQR_FrRateLimitDec_Nm] -> TorqueModule/105(VTQR_FrRateLimitDec_Nm)
  [VTQR_RrRateLimitInc_Nm] -> TorqueModule/106(VTQR_RrRateLimitInc_Nm)
  [VTQR_RrRateLimitDec_Nm] -> TorqueModule/107(VTQR_RrRateLimitDec_Nm)
  [VTQD_CreepTCSActive_flg] -> Signal_convert/97(VTQD_CreepTCSActive_flg)
  TorqueModule/69(VTQD_CreepTCSActive_flg) -> [VTQD_CreepTCSActive_flg]
  [VINP_RrPTCSActive_flg] -> Signal_convert/98(VINP_RrPTCSActive_flg)
  [VINP_FrPTCSActive_flg] -> Signal_convert/99(VINP_FrPTCSActive_flg)
  [VINP_FrMCUDCBusVolt_V] -> TorqueModule/108(VINP_FrMCUDCBusVolt_V)
  [VINP_RrMCUDCBusVolt_V] -> TorqueModule/109(VINP_RrMCUDCBusVolt_V)
  VINP_RrMCUDCBusVolt_V/1 -> [VINP_RrMCUDCBusVolt_V]
  VINP_FrMCUDCBusVolt_V/1 -> [VINP_FrMCUDCBusVolt_V]
  Signal_convert/50(VTQD_SkipDirect_enum) -> [VTQD_SkipDirect_enum]
  Signal_convert/49(VTQD_ActWhlSkipSta_enum) -> [VTQD_ActWhlSkipSta_enum]
  [VTQD_ActWhlSkipSta_enum] -> TorqueModule/110(VTQD_ActWhlSkipSta_enum)
  [VTQD_SkipDirect_enum] -> TorqueModule/111(VTQD_SkipDirect_enum)
  [VTQD_EPBCarWashMode_flg] -> VTQD_EPBCarWashMode_flg/1
  VDDM_ESC5Err_flg/1 -> [VDDM_ESC5Err_flg]
  VDDM_EPB1Err_flg/1 -> [VDDM_EPB1Err_flg]
  VDDM_EPBSigErrCFS_flg/1 -> [VDDM_EPBSigErrCFS_flg]
  VDDM_ESC1Err_flg/1 -> [VDDM_ESC1Err_flg]
  VDDM_VCURAPSErrLv2_flg/1 -> [VDDM_VCURAPSErrLv2_flg]
  VDDM_VCURAPSErrLv3_flg/1 -> [VDDM_VCURAPSErrLv3_flg]
  VINP_APSStaSystem_enum/1 -> [VINP_APSStaSystem_enum]
  [VDDM_VCURAPSErrLv2_flg] -> ShiftModule/24(VDDM_VCURAPSErrLv2_flg)
  [VDDM_VCURAPSErrLv3_flg] -> ShiftModule/25(VDDM_VCURAPSErrLv3_flg)
  [VINP_APSStaSystem_enum] -> ShiftModule/26(VINP_APSStaSystem_enum)
  [VDDM_EPBSigErrCFS_flg] -> TorqueModule/115(VDDM_EPBSigErrCFS_flg)
  VINP_FrTMTemp_C/1 -> [VINP_FrTMTemp_C]
  VINP_RrTMTemp_C/1 -> [VINP_RrTMTemp_C]
  VINP_FrMCUTemp_C/1 -> [VINP_FrMCUTemp_C]
  VINP_RrMCUTemp_C/1 -> [VINP_RrMCUTemp_C]
  [VINP_FrMCUTemp_C] -> TorqueModule/116(VINP_FrMCUTemp_C)
  [VINP_FrTMTemp_C] -> TorqueModule/117(VINP_FrTMTemp_C)
  [VINP_RrMCUTemp_C] -> TorqueModule/118(VINP_RrMCUTemp_C)
  [VINP_RrTMTemp_C] -> TorqueModule/119(VINP_RrTMTemp_C)
  VINP_ADASAEBSta_enum/1 -> [VINP_ADASAEBSta_enum]
  [VINP_ADASAEBSta_enum] -> TorqueModule/120(VINP_ADASAEBSta_enum)
  [VINP_VehicleType_enum] -> Signal_convert/100(VINP_VehicleType_enum)
  [VINP_IVIEscapeModeCmd_flg] -> Signal_convert/101(VINP_IVIEscapeModeCmd_flg)
  Signal_convert/51(VTQD_IVIRockModeEn_flg) -> VTQD_IVIRockModeEn_flg/1, [VTQD_IVIRockModeEn_flg]
  [VTQD_FrShaftSpd_rpm] -> ShiftModule/27(VTQD_FrShaftSpd_rpm)
  [VTQD_RrShaftSpd_rpm] -> ShiftModule/28(VTQD_RrShaftSpd_rpm)
  Signal_convert/52(VTQD_SimSouWaveReq_pct) -> VTQD_SimSouWaveReq_pct/1
  VINP_ESCOFFStatus_enum/1 -> [VINP_ESCOFFStatus_enum]
  [VINP_ESCOFFStatus_enum] -> Signal_convert/102(VINP_ESCOFFStatus_enum)
  TorqueModule/70(VTQD_EscapModeTqLim_flg) -> [VTQD_EscapModeTqLim_flg]
  [VTQD_EscapModeTqLim_flg] -> Signal_convert/103(VTQD_EscapModeTqLim_flg)
  Signal_convert/53(VTQD_RockModeTCSReq_flg) -> VTQD_RockModeTCSReq_flg/1
  [VTQD_CoordWhlTqDemFr_Nm] -> Signal_convert/104(VTQD_CoordWhlTqDemFr_Nm)
  [VTQD_CoordWhlTqDemRr_Nm] -> Signal_convert/105(VTQD_CoordWhlTqDemRr_Nm)
  [VTQD_WhlTqCapGenFr_Nm] -> Signal_convert/106(VTQD_WhlTqCapGenFr_Nm)
  [VTQD_WhlTqCapGenRr_Nm] -> Signal_convert/107(VTQD_WhlTqCapGenRr_Nm)
  [VTQR_FrTqZeroTransLowBound_Nm] -> TorqueModule/121(VTQR_FrTqZeroTransLowBound_Nm)
  [VTQR_RrTqZeroTransUpBound_Nm] -> TorqueModule/122(VTQR_RrTqZeroTransUpBound_Nm)
  VTQR_RrTqZeroTransUpBound_Nm/1 -> [VTQR_RrTqZeroTransUpBound_Nm]
  VTQR_FrTqZeroTransLowBound_Nm/1 -> [VTQR_FrTqZeroTransLowBound_Nm]
  TorqueModule/71(VTQD_TMEnOutpTqSta_enum) -> VTQD_TMEnOutpTqSta_enum/1
  [VDDM_EPB1Err_flg] -> TorqueModule/112(VDDM_EPB1Err_flg)
  [VDDM_ESC1Err_flg] -> TorqueModule/113(VDDM_ESC1Err_flg)
  [VDDM_ESC5Err_flg] -> TorqueModule/114(VDDM_ESC5Err_flg)
  VDDM_VehMalfunLevel_enum/1 -> [VDDM_VehMalfunLevel_enum]
  VDDM_MCUR1Err_flg/1 -> [VDDM_MCUR1Err_flg]
  VDDM_ShifterSigErrCFS_flg/1 -> [VDDM_ShifterSigErrCFS_flg]
  VDDM_Shifter1Err_flg/1 -> [VDDM_Shifter1Err_flg]
  VDDM_MCUF1Err_flg/1 -> [VDDM_MCUF1Err_flg]
  VDDM_RegenErrCFS_flg/1 -> [VDDM_RegenErrCFS_flg]
  VDDM_4D2CErr_flg/1 -> [VDDM_4D2CErr_flg]
  [VDDM_VehMalfunLevel_enum] -> TorqueModule/123(VDDM_VehMalfunLevel_enum)
  [VDDM_MCUF1Err_flg] -> TorqueModule/124(VDDM_MCUF1Err_flg)
  [VDDM_MCUR1Err_flg] -> TorqueModule/125(VDDM_MCUR1Err_flg)
  [VDDM_Shifter1Err_flg] -> TorqueModule/126(VDDM_Shifter1Err_flg)
  [VDDM_ShifterSigErrCFS_flg] -> TorqueModule/127(VDDM_ShifterSigErrCFS_flg)
  [VDDM_4D2CErr_flg] -> TorqueModule/128(VDDM_4D2CErr_flg)
  [VDDM_RegenErrCFS_flg] -> TorqueModule/129(VDDM_RegenErrCFS_flg)
  Signal_convert/54(VTQD_ShifterHandleCmd_enum) -> [VTQD_ShifterHandleCmd_enum]
  Signal_convert/55(VTQD_ShifterFailsta_enum) -> [VTQD_ShifterFailsta_enum]
  Signal_convert/56(SWC_RegenUp) -> [SWC_RegenUp]
  Signal_convert/57(SWC_RegenDown) -> [SWC_RegenDown]
  [VINP_ShifterHandleCmd_enum] -> Signal_convert/108(VINP_ShifterHandleCmd_enum)
  [VDDM_Shifter1Err_flg] -> Signal_convert/110(VDDM_Shifter1Err_flg)
  VINP_ShifterFailsta_enum/1 -> [VINP_ShifterFailsta_enum]
  [VINP_ShifterFailsta_enum] -> Signal_convert/109(VINP_ShifterFailsta_enum)
  [VDDM_Shifter1Err_flg] -> ShiftModule/29(VDDM_Shifter1Err_flg)
  [SWC_RegenUp] -> ShiftModule/30(SWC_RegenUp)
  [SWC_RegenDown] -> ShiftModule/31(SWC_RegenDown)
  [VDDM_ShifterSigErrCFS_flg] -> ShiftModule/32(VDDM_ShifterSigErrCFS_flg)
  [VTQD_ShifterFailsta_enum] -> ShiftModule/33(VTQD_ShifterFailsta_enum)
  Signal_convert/58(VTQD_SimSoundCmd_pct) -> [VTQD_SimSoundCmd_pct]  "VTQD_SimSoundCmd_pct"
  ShiftModule/8(VTQD_ForceP_flg) -> VTQD_ForceP_flg/1
  TorqueModule/72(VTQD_SlideRegenLimTq_Nm) -> VTQD_SlideRegenLimTq_Nm/1
  [VTQD_SimSoundCmd_pct] -> VTQD_SimSoundCmd_pct/1
  [VDDM_VCURAPSErrLv2_flg] -> TorqueModule/130(VDDM_VCURAPSErrLv2_flg)
  [VINP_EPBSta_enum] -> ShiftModule/34(VINP_EPBSta_enum)
